simulink model "cams"  (R2024a)
settings: Solver=VariableStepAuto  StartTime=0.0  StopTime=5  RelTol=1e-3
values from neighbouring files (symbols this model uses):
  N = 2    [cams2.m]    (also in ftc_2AGENTS.m; ftc_4AGENTS.m = 4)
undefined symbols (not defined in the file or in its folder): param
settings Model: Creator=antor  LastModifiedBy=antor

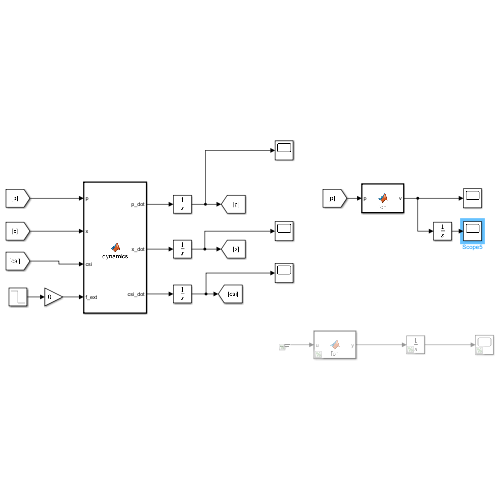
[thumbnail: Simulink's stored preview of the top-level diagram]
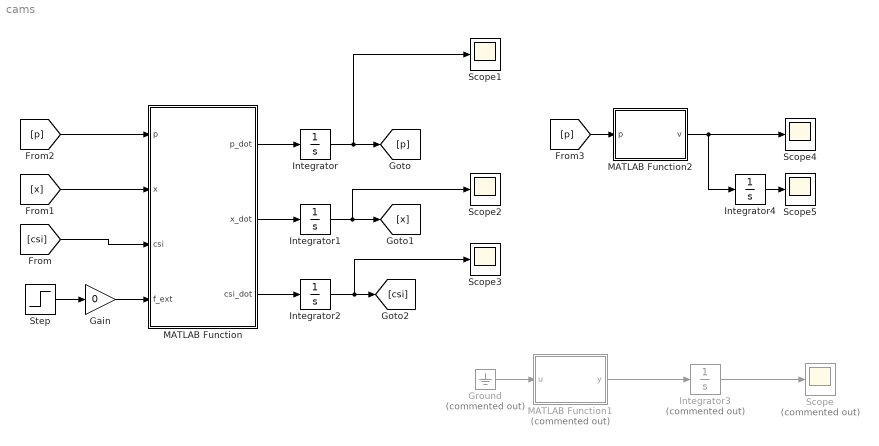
== system cams ==
  Gain : Gain  Gain=0
  Ground : Ground  Commented=on
  Integrator : Integrator  InitialCondition=zeros(3, param.N)
  Integrator1 : Integrator  InitialCondition=100*ones(1, param.N)
  Integrator2 : Integrator  InitialCondition=2*ones(3, nchoosek(param.N, 2))
  Integrator3 : Integrator  Commented=on  InitialCondition=zeros(3, N)
  Integrator4 : Integrator  InitialCondition=[1, -1; 1, -1; 1, -1]
  MATLAB Function : MATLAB Function  TreatAsAtomicUnit=on
  MATLAB Function1 : MATLAB Function  Commented=on  TreatAsAtomicUnit=on
  MATLAB Function2 : MATLAB Function  TreatAsAtomicUnit=on
  Scope : Scope  Commented=on
  Scope{1..5} (5 alike) : Scope
  Step : Step  Time=10  Before=[2; 2; 2]  After=[0; 0; 0]  SampleTime=0
  wires:
  MATLAB Function/1(p_dot) -> Integrator/1
  MATLAB Function/2(x_dot) -> Integrator1/1
  MATLAB Function/3(csi_dot) -> Integrator2/1
  Integrator2/1 -> Scope3/1, [csi]
  Integrator1/1 -> Scope2/1, [x]
  Integrator/1 -> Scope1/1, [p]
  [csi] -> MATLAB Function/3(csi)
  [x] -> MATLAB Function/2(x)
  [p] -> MATLAB Function/1(p)
  Step/1 -> Gain/1
  MATLAB Function1/1(y) -> Integrator3/1
  Integrator3/1 -> Scope/1
  Ground/1 -> MATLAB Function1/1(u)
  [p] -> MATLAB Function2/1(p)
  MATLAB Function2/1(v) -> Integrator4/1, Scope4/1
  Integrator4/1 -> Scope5/1
  Gain/1 -> MATLAB Function/4(f_ext)

== matlab function cams/MATLAB Function1 ==
  data: u input; y output
function y = fcn(u)
    y = zeros(3, 5);
end

== matlab function cams/MATLAB Function ==
  data: p input; p_dot output; x input; csi input; f_ext input; x_dot output; csi_dot output; param parameter
function [p_dot, x_dot, csi_dot] = dynamics(p, x, csi, f_ext, param)
    N = param.N;
    N = 2;
    E = param.E;
    K = param.K;
    M = param.M;
    B = param.B;

    p_dot = zeros(3, N);
    x_dot = zeros(1, N);
    csi_dot = zeros(3, nchoosek(N, 2));
    r = zeros(1, 3, N);
    h = zeros(1, 3, N, nchoosek(N, 2));

    x = x';

    for i = 1:N
        r(:, :, i) = (B(:, :, i)*M(:, :, i)\p(:, i)).'./repmat(x(:, i), 1, 3);
        for j = 1:nchoosek(N, 2)
            % h(:, :, i, j) = x(:, i)*(K(:, :, j)*csi(:, j)).';
        end
    end

    for i = 1:N
        p_dot(:, i) = - r(:, :, i).'*x(:, i);
        x_dot(:, i) = r(:, :, i)*(M(:, :, i)\p(:, i));
        for j = 1:nchoosek(N, 2)
            p_dot(:, i) = p_dot(:, i) + E(i, j)*ones(1, 3)*K(:, :, j)*csi(:, j);
            x_dot(:, i) = x_dot(:, i) - h(:, :, i, j)*K(:, :, j)*csi(:, j);
            csi_dot(:, j) = csi_dot(:, j) - E(i, j)*(M(:, :, i)\p(:, i)) + h(:, :, i, j).'.*repmat(x(:, i), 3, 1);
        end
    end
    p_dot(:, 1) = p_dot(:, 1) + f_ext;

end

== matlab function cams/MATLAB Function2 ==
  data: v output; p input; param parameter
function v = fcn(p, param)
    N = param.N;
    N = 2;
    M = param.M;

    v = zeros(3, N);
    for i = 1:N
        v(:, i) = M(:, :, i)\p(:, i);
    end
end
